simulink library "Driver_Override_vx_Obstacle"  (R2025b)
settings: Solver=VariableStepAuto  StartTime=0.0  StopTime=10.0  RelTol=1e-3
undefined symbols (not defined in the file): Scene
libraries: Object_Traffic_Light x2
Description:
  | Simscape Vehicle Templates Library
  | 
  | Copyright 2018-2025 The MathWorks, Inc.
settings Model: Creator=smiller  LastModifiedBy=smiller
settings OptimizationCC: ReuseModelBlockBuffer=off
settings ModelReferenceCC: EnableRefExpFcnMdlSchedulingChecks=on
settings RTWCC: GPUComputeCapability=3.5

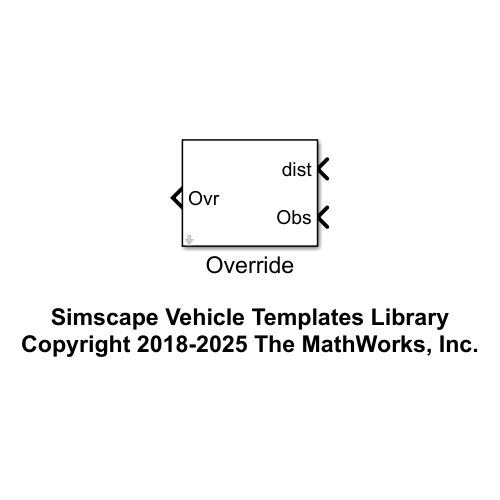
[thumbnail: Simulink's stored preview of the top-level diagram]
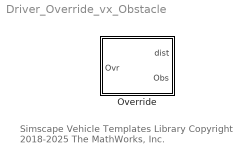
== system Driver_Override_vx_Obstacle ==
  note: Simscape Vehicle Templates Library
      | Copyright 2018-2025 The MathWorks, Inc.
  Override : Subsystem  mask(Driver Override Two Traffic Lights){override=Scene.Mallory_Park_Obstacle.Override}
      mask prompts: override "Override parameters (structure)"
      mask help: Models logic to override driver commands based on two traffic lights.

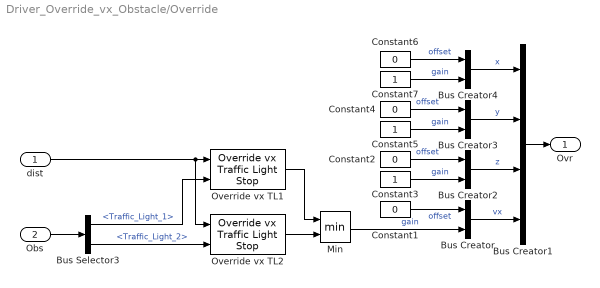
== system Driver_Override_vx_Obstacle/Override ==
  dist : Inport
  Obs : Inport  Port=2
  Bus Creator{,2..4} (4 alike) : BusCreator  Inputs=2
  Bus Creator1 : BusCreator  Inputs=4
  Bus Selector3 : BusSelector  OutputSignals=Traffic_Light_1,Traffic_Light_2
  Constant{1..2,4,6} (4 alike) : Constant  Value=0
  Constant3 : Constant
  Constant5 : Constant
  Constant7 : Constant
  Min : MinMax  Inputs=2  ZeroCross=off
  Override vx TL1 : Object_Traffic_Light/Override vx Traffic Light Stop  x_start=override.vx.TL1.d_start  x_end=override.vx.TL1.d_end  t_to_min=override.vx.TL1.t_to_min  t_to_max=override.vx.TL1.t_to_max
  Override vx TL2 : Object_Traffic_Light/Override vx Traffic Light Stop  x_start=override.vx.TL2.d_start  x_end=override.vx.TL2.d_end  t_to_min=override.vx.TL2.t_to_min  t_to_max=override.vx.TL2.t_to_max
  Ovr : Outport  VectorParamsAs1DForOutWhenUnconnected=off
  wires:
  Bus Selector3/2 -> Override vx TL2/2  "<Traffic_Light_2>"
  Override vx TL1/1 -> Min/1
  Bus Selector3/1 -> Override vx TL1/2  "<Traffic_Light_1>"
  Obs/1 -> Bus Selector3/1
  Override vx TL2/1 -> Min/2
  dist/1 -> Override vx TL2/1, Override vx TL1/1
  Bus Creator1/1 -> Ovr/1
  Constant1/1 -> Bus Creator/1  "offset"
  Min/1 -> Bus Creator/2  "gain"
  Constant6/1 -> Bus Creator4/1  "offset"
  Constant7/1 -> Bus Creator4/2  "gain"
  Constant5/1 -> Bus Creator3/2  "gain"
  Constant4/1 -> Bus Creator3/1  "offset"
  Constant3/1 -> Bus Creator2/2  "gain"
  Bus Creator2/1 -> Bus Creator1/3  "z"
  Constant2/1 -> Bus Creator2/1  "offset"
  Bus Creator3/1 -> Bus Creator1/2  "y"
  Bus Creator/1 -> Bus Creator1/4  "vx"
  Bus Creator4/1 -> Bus Creator1/1  "x"
